simulink model "STH_Linear"  (R2020b)
settings: Solver=FixedStepAuto  StartTime=0.0  StopTime=1800  FixedStep=5  RelTol=1e-3
values from neighbouring files (symbols this model uses):
  A = [A11, A12; A21, A22]    [Exp2_STH.m]
  B = horzcat(Bu, Bd)    [Exp2_STH.m]
  C = [1, 0]    [Exp2_STH.m]
  D = [0, 0, 0, 0]    [Exp2_STH.m]
  Ts = 51.67    [Exp2_STH.m]
settings Model: Creator=franc  LastModifiedBy=franc

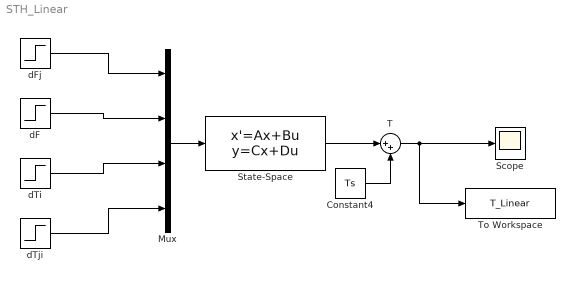
== system STH_Linear ==
  "            T" : Sum  Inputs=|++
  Constant4 : Constant  Value=Ts
  Mux : Mux
  Scope : Scope
  State-Space : StateSpace  A=A  B=B  C=C  D=D  InitialCondition=0
  To Workspace : ToWorkspace  VariableName=T_Linear  SaveFormat=Timeseries  SampleTime=-1
  dF : Step  Time=0  After=0  SampleTime=0
  dFj : Step  Time=0  After=4.72e-5  SampleTime=0
  dTi : Step  Time=0  After=0  SampleTime=0
  dTji : Step  Time=0  After=0  SampleTime=0
  wires:
  Mux/1 -> State-Space/1
  dF/1 -> Mux/2
  dTi/1 -> Mux/3
  dTji/1 -> Mux/4
  dFj/1 -> Mux/1
  "            T"/1 -> Scope/1, To Workspace/1
  State-Space/1 -> "            T"/1
  Constant4/1 -> "            T"/2
